simulink model "NN Controlled IM Drive"  (R2020b)
settings: Solver=ode4  StartTime=0.0  StopTime=5  RelTol=1e-3
InitFcn:
  | %clear;
  | %clc;
  | 
  | %Motor Parameters
  | r1 = 1.405;
  | l1  = 0.005839;
  | r2 = 1.395;
  | l2 = 0.005839;
  | Lm = 0.1722;
  | J = 0.0131;
  | 
  | %Motor Rated Values
  | Vrat = 400;
  | frat = 50;
  | 
  | x1 = 2*pi*frat*l1;
  | x2 = 2*pi*frat*l2;
  | Xm = 2*pi*frat*Lm;
  | Prat = 4*1000;
  | Nrat = 1430;
  | P = 4;
  | Ns = 120*frat/P;
  | nrat = Nrat*2*pi/60;
  | ns = Ns*2*pi/60;
  | srat = (Ns-Nrat)/Ns;
  | 
  | E1 = Vrat/sqrt(3); %phase voltage
  | IL = E1/( (r1 + (1i*x1) ) + ( ( (1i*x2) +(r2/srat) )*1i*Xm / ( (1i*Xm) + (1i*x2) + (r2/srat) ) ) );
  | E2 = E1 - (IL*(r1 + (1i*x1) ) );
  | Trat = (3/(ns))*srat*abs(E2)*abs(E2)*r2/((r2*r2) + (srat*srat*x2*x2));
  | %Trat = Prat/nrat;
  | 
  | %System Variables
  | Tsys = (1e-6);
  | Ts = (100e-6);
  | freq = 50;
  | ws = freq*2*pi;
  | 
  | m=1*freq/50;
  | %m = 1 * (freq/50);
  | Vbus = (400*sqrt(2)*2/sqrt(3)) / (1.15);
  | 
  | Vref = (Vbus*sqrt(3)/2) * m;
  | delay = Ts/Tsys;
  | 
  | % Motor Starting Parameters
  | inc_time = 0.1;
  | 
  | %Motor Loading time
  | load_time = 0;
  | 
  | %No. of Hybrid Zones
  | numzones = 3;
  | 
  | %Load ML model Weights
  | 
  | W1R_s1 = readmatrix('Regression Weights\W1_subnet1_tmp_odd_90.xlsx');
  | b1R_s1 = readmatrix('Regression Weights\b1_subnet1_tmp_odd_90.xlsx');
  | W1R_s2 = readmatrix('Regression Weights\W1_subnet2_tmp_odd_90.xlsx');
  | b1R_s2 = readmatrix('Regression Weights\b1_subnet2_tmp_odd_90.xlsx');
  | ... (+47 lines)
undefined symbols (not defined in the file): DiscIntNeverNeededParam
libraries: powerlib x22, simulink x20, pid_lib x4, powerlib_meascontrol x3, simulink_extras x2
(part 2 of 3)

== system NN Controlled IM Drive/Space Vector PWM based VSI /Gating Pulse Generator/Gate Pulse Generator for 1012 Sequence ==
  "S1, S3, S5, sector" : Inport
  AND{,1..5} (6 alike) : Logic  IconShape=distinctive  AllPortsSameDT=off  OutDataTypeStr=boolean
  Constant : Constant  Value=2
  Data Type Conversion : DataTypeConversion
  Demux : Demux
  For Even Sector : Subsystem
  For Odd Sector : Subsystem
  Mod : Math  Operator=mod  SaturateOnIntegerOverflow=on
  Mux : Mux  Inputs=3
  NOT : Logic  Operator=NOT  IconShape=distinctive  AllPortsSameDT=off  OutDataTypeStr=boolean
  OR : Logic  Operator=OR  IconShape=distinctive  AllPortsSameDT=off  OutDataTypeStr=boolean
  OR1 : Logic  Operator=OR  IconShape=distinctive  AllPortsSameDT=off  OutDataTypeStr=boolean
  OR2 : Logic  Operator=OR  IconShape=distinctive  AllPortsSameDT=off  OutDataTypeStr=boolean
  Scope1 : Scope  NumInputPorts=4
  Gate 1 Pulse : Outport
  Gate 3 Pulse : Outport  Port=2
  Gate 5 Pulse : Outport  Port=3
  wires:
  For Odd Sector/3(Gate 5 Pulse) -> AND5/1
  For Odd Sector/1(Gate 1 Pulse) -> AND3/1
  For Even Sector/3(Gate 5 Pulse) -> AND2/1
  For Even Sector/2(Gate 3 Pulse) -> AND1/1
  OR2/1 -> Scope1/3, Gate 5 Pulse/1
  OR1/1 -> Scope1/2, Gate 3 Pulse/1
  Demux/3 -> Mux/3
  For Even Sector/1(Gate 1 Pulse) -> AND/1
  AND4/1 -> OR1/1
  OR/1 -> Scope1/1, Gate 1 Pulse/1
  AND5/1 -> OR2/1
  Demux/2 -> Mux/2
  AND1/1 -> OR1/2
  AND/1 -> OR/2
  Mod/1 -> Data Type Conversion/1
  Demux/4 -> Scope1/4, Mod/1
  Data Type Conversion/1 -> AND3/2, AND4/2, AND5/2, NOT/1
  AND2/1 -> OR2/2
  Demux/1 -> Mux/1
  Mux/1 -> For Even Sector/1("S1, S3, S1"), For Odd Sector/1("S1, S3, S5")
  Constant/1 -> Mod/2
  NOT/1 -> AND/2, AND1/2, AND2/2
  For Odd Sector/2(Gate 3 Pulse) -> AND4/1
  "S1, S3, S5, sector"/1 -> Demux/1
  AND3/1 -> OR/1

== system NN Controlled IM Drive/Space Vector PWM based VSI /Gating Pulse Generator/Gate Pulse Generator for 2721 Sequence ==
  "S1, S3, S5, sector" : Inport
  AND{,1..5} (6 alike) : Logic  IconShape=distinctive  AllPortsSameDT=off  OutDataTypeStr=boolean
  Constant : Constant  Value=2
  Data Type Conversion : DataTypeConversion
  Demux : Demux
  For Even Sector : Subsystem
  For Odd Sector : Subsystem
  Mod : Math  Operator=mod  SaturateOnIntegerOverflow=on
  Mux : Mux  Inputs=3
  NOT : Logic  Operator=NOT  IconShape=distinctive  AllPortsSameDT=off  OutDataTypeStr=boolean
  OR : Logic  Operator=OR  IconShape=distinctive  AllPortsSameDT=off  OutDataTypeStr=boolean
  OR1 : Logic  Operator=OR  IconShape=distinctive  AllPortsSameDT=off  OutDataTypeStr=boolean
  OR2 : Logic  Operator=OR  IconShape=distinctive  AllPortsSameDT=off  OutDataTypeStr=boolean
  Scope1 : Scope  NumInputPorts=4
  Gate 1 Pulse : Outport
  Gate 3 Pulse : Outport  Port=2
  Gate 5 Pulse : Outport  Port=3
  wires:
  For Odd Sector/3(Gate 5 Pulse) -> AND5/1
  For Odd Sector/1(Gate 1 Pulse) -> AND3/1
  For Even Sector/3(Gate 5 Pulse) -> AND2/1
  OR2/1 -> Scope1/3, Gate 5 Pulse/1
  For Even Sector/2(Gate 3 Pulse) -> AND1/1
  OR1/1 -> Scope1/2, Gate 3 Pulse/1
  Demux/3 -> Mux/3
  AND4/1 -> OR1/1
  OR/1 -> Scope1/1, Gate 1 Pulse/1
  AND5/1 -> OR2/1
  Demux/2 -> Mux/2
  For Odd Sector/2(Gate 3 Pulse) -> AND4/1
  AND1/1 -> OR1/2
  AND/1 -> OR/2
  Mod/1 -> Data Type Conversion/1
  Data Type Conversion/1 -> AND3/2, AND4/2, AND5/2, NOT/1
  AND2/1 -> OR2/2
  "S1, S3, S5, sector"/1 -> Demux/1
  AND3/1 -> OR/1
  Demux/4 -> Scope1/4, Mod/1
  Demux/1 -> Mux/1
  Mux/1 -> For Even Sector/1("S1, S3, S5"), For Odd Sector/1("S1, S3, S1")
  Constant/1 -> Mod/2
  NOT/1 -> AND/2, AND1/2, AND2/2
  For Even Sector/1(Gate 1 Pulse) -> AND/1

== system NN Controlled IM Drive/Space Vector PWM based VSI /Gating Pulse Generator/Gate Pulse Generator for 7212 Sequence ==
  "S1, S3, S5, sector" : Inport
  AND{,1..5} (6 alike) : Logic  IconShape=distinctive  AllPortsSameDT=off  OutDataTypeStr=boolean
  Constant : Constant  Value=2
  Data Type Conversion : DataTypeConversion
  Demux : Demux
  For Even Sector : Subsystem
  For Odd Sector : Subsystem
  Mod : Math  Operator=mod  SaturateOnIntegerOverflow=on
  Mux : Mux  Inputs=3
  NOT : Logic  Operator=NOT  IconShape=distinctive  AllPortsSameDT=off  OutDataTypeStr=boolean
  OR : Logic  Operator=OR  IconShape=distinctive  AllPortsSameDT=off  OutDataTypeStr=boolean
  OR1 : Logic  Operator=OR  IconShape=distinctive  AllPortsSameDT=off  OutDataTypeStr=boolean
  OR2 : Logic  Operator=OR  IconShape=distinctive  AllPortsSameDT=off  OutDataTypeStr=boolean
  Scope1 : Scope  NumInputPorts=4
  Gate 1 Pulse : Outport
  Gate 3 Pulse : Outport  Port=2
  Gate 5 Pulse : Outport  Port=3
  wires:
  For Odd Sector/3(Gate 5 Pulse) -> AND5/1
  For Odd Sector/1(Gate 1 Pulse) -> AND3/1
  For Even Sector/3(Gate 5 Pulse) -> AND2/1
  For Even Sector/2(Gate 3 Pulse) -> AND1/1
  OR2/1 -> Scope1/3, Gate 5 Pulse/1
  OR1/1 -> Scope1/2, Gate 3 Pulse/1
  Demux/3 -> Mux/3
  For Even Sector/1(Gate 1 Pulse) -> AND/1
  AND4/1 -> OR1/1
  OR/1 -> Scope1/1, Gate 1 Pulse/1
  AND5/1 -> OR2/1
  Demux/2 -> Mux/2
  AND1/1 -> OR1/2
  AND/1 -> OR/2
  Mod/1 -> Data Type Conversion/1
  Demux/4 -> Scope1/4, Mod/1
  Data Type Conversion/1 -> AND3/2, AND4/2, AND5/2, NOT/1
  AND2/1 -> OR2/2
  Demux/1 -> Mux/1
  Mux/1 -> For Even Sector/1("S1, S3, S1"), For Odd Sector/1("S1, S3, S5")
  Constant/1 -> Mod/2
  NOT/1 -> AND/2, AND1/2, AND2/2
  For Odd Sector/2(Gate 3 Pulse) -> AND4/1
  "S1, S3, S5, sector"/1 -> Demux/1
  AND3/1 -> OR/1

== system NN Controlled IM Drive/Space Vector PWM based VSI /Switching Times and Sector/Angle Calculation1 ==
  freq : Inport
  Delay : Delay  DelayLength=1  InitialCondition=0  UseCircularBuffer=on
  Gain1 : Gain  Gain=Tsys
  MATLAB Function : MATLAB Function  TreatAsAtomicUnit=on
  Scope : Scope
  Zero-Order Hold : ZeroOrderHold  SampleTime=Ts
  w : Gain  Gain=2*pi
  Angle : Outport
  tag scope: wt=global
  wires:
  freq/1 -> w/1, Scope/1
  Gain1/1 -> MATLAB Function/2(wTs)
  Zero-Order Hold/1 -> Angle/1
  Delay/1 -> MATLAB Function/1(wold)
  MATLAB Function/1(wnew) -> Delay/1, Zero-Order Hold/1, [wt]
  w/1 -> Gain1/1

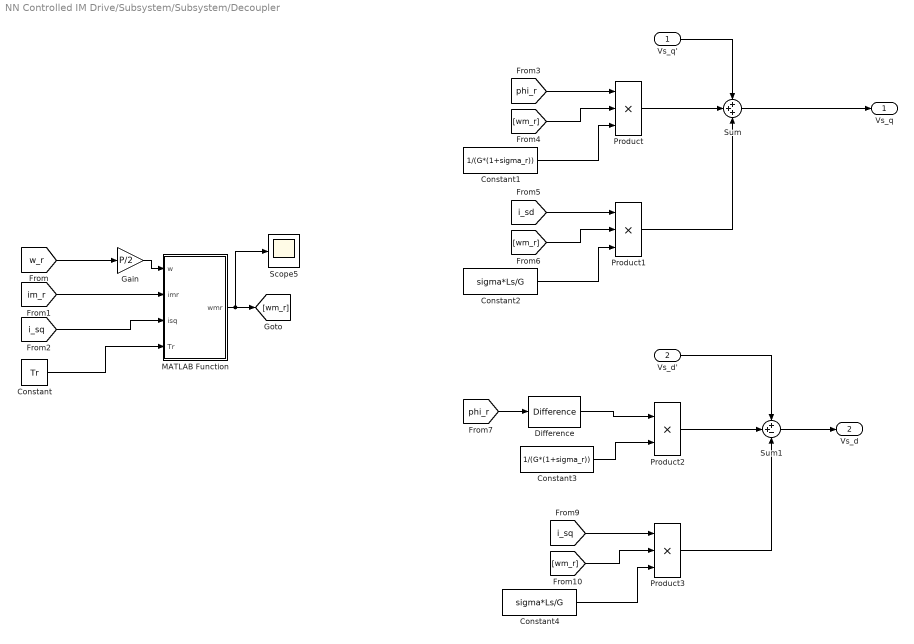
== system NN Controlled IM Drive/Subsystem/Subsystem/Decoupler ==
  Vs_q' : Inport
  Vs_d' : Inport  Port=2
  Constant : Constant  Value=Tr
  Constant1 : Constant  Value=1/(G*(1+sigma_r))
  Constant2 : Constant  Value=sigma*Ls/G
  Constant3 : Constant  Value=1/(G*(1+sigma_r))
  Constant4 : Constant  Value=sigma*Ls/G
  Difference : simulink/Discrete/Difference  ICPrevInput=0.0  OutMin=[]  OutMax=[]  OutDataType=fixdt(1, 16)  OutScaling=2^-10  DoSatur=off
  Gain : Gain  Gain=P/2
  MATLAB Function : MATLAB Function  TreatAsAtomicUnit=on
  Product : Product  Inputs=3
  Product1 : Product  Inputs=3
  Product2 : Product
  Product3 : Product  Inputs=3
  Scope5 : Scope
  Sum : Sum  Inputs=+++
  Sum1 : Sum  Inputs=++-
  Vs_q : Outport
  Vs_d : Outport  Port=2
  wires:
  [im_r] -> MATLAB Function/2(imr)
  [i_sq] -> MATLAB Function/3(isq)
  Constant/1 -> MATLAB Function/4(Tr)
  MATLAB Function/1(wmr) -> Scope5/1, [wm_r]
  [phi_r] -> Product/1
  [wm_r] -> Product/2
  Constant1/1 -> Product/3
  Vs_q'/1 -> Sum/1
  Product/1 -> Sum/2
  Constant2/1 -> Product1/3
  [wm_r] -> Product1/2
  [i_sd] -> Product1/1
  Product1/1 -> Sum/3
  Sum/1 -> Vs_q/1
  Product3/1 -> Sum1/3
  [i_sq] -> Product3/1
  [wm_r] -> Product3/2
  Constant4/1 -> Product3/3
  Difference/1 -> Product2/1
  Vs_d'/1 -> Sum1/1
  Sum1/1 -> Vs_d/1
  [phi_r] -> Difference/1
  Constant3/1 -> Product2/2
  [w_r] -> Gain/1
  Gain/1 -> MATLAB Function/1(w)
  Product2/1 -> Sum1/2

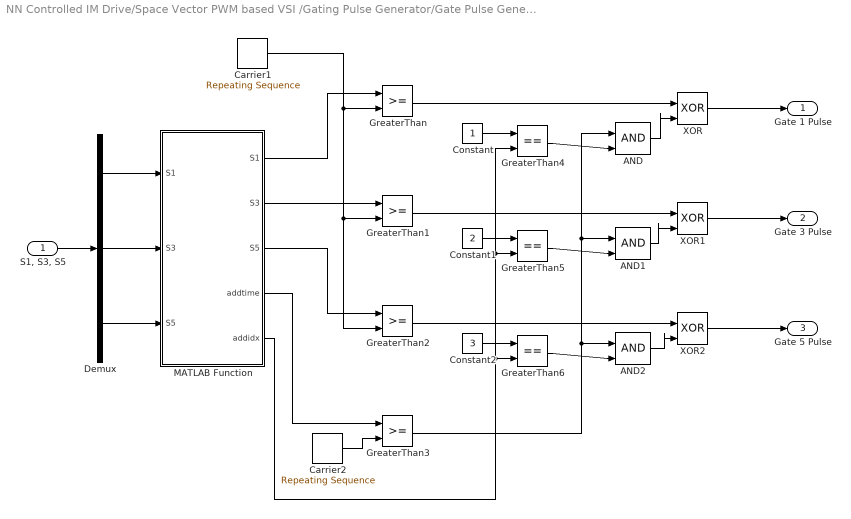
== system NN Controlled IM Drive/Space Vector PWM based VSI /Gating Pulse Generator/Gate Pulse Generator for 0121 Sequence/For Even Sector ==
  "S1, S3, S5" : Inport
  AND : Logic  IconShape=distinctive  AllPortsSameDT=off  OutDataTypeStr=boolean
  AND1 : Logic  IconShape=distinctive  AllPortsSameDT=off  OutDataTypeStr=boolean
  AND2 : Logic  IconShape=distinctive  AllPortsSameDT=off  OutDataTypeStr=boolean
  Carrier1 : simulink/Sources/Repeating Sequence  rep_seq_t=[0 Ts/2 Ts]  rep_seq_y=[0 Ts-(1e-16) 0]
  Carrier2 : simulink/Sources/Repeating Sequence  rep_seq_t=[0 Ts/2 Ts]  rep_seq_y=[Ts-(1e-16) 0 Ts-(1e-16)]
  Constant : Constant
  Constant1 : Constant  Value=2
  Constant2 : Constant  Value=3
  Demux : Demux  Outputs=3
  GreaterThan{,1..3} (4 alike) : RelationalOperator  OutDataTypeStr=boolean  RndMeth=Simplest
  GreaterThan4 : RelationalOperator  Operator===  OutDataTypeStr=boolean  RndMeth=Simplest
  GreaterThan5 : RelationalOperator  Operator===  OutDataTypeStr=boolean  RndMeth=Simplest
  GreaterThan6 : RelationalOperator  Operator===  OutDataTypeStr=boolean  RndMeth=Simplest
  MATLAB Function : MATLAB Function  TreatAsAtomicUnit=on
  XOR : Logic  Operator=XOR  IconShape=distinctive  AllPortsSameDT=off  OutDataTypeStr=boolean
  XOR1 : Logic  Operator=XOR  IconShape=distinctive  AllPortsSameDT=off  OutDataTypeStr=boolean
  XOR2 : Logic  Operator=XOR  IconShape=distinctive  AllPortsSameDT=off  OutDataTypeStr=boolean
  Gate 1 Pulse : Outport
  Gate 3 Pulse : Outport  Port=2
  Gate 5 Pulse : Outport  Port=3
  wires:
  Demux/3 -> MATLAB Function/3("S5 ")
  Demux/1 -> MATLAB Function/1("S1 ")
  "S1, S3, S5"/1 -> Demux/1
  Demux/2 -> MATLAB Function/2("S3 ")
  MATLAB Function/5(addidx) -> GreaterThan6/2, GreaterThan5/2, GreaterThan4/2
  Constant1/1 -> GreaterThan5/1
  Constant/1 -> GreaterThan4/1
  XOR1/1 -> Gate 3 Pulse/1
  GreaterThan6/1 -> AND2/2
  Constant2/1 -> GreaterThan6/1
  GreaterThan5/1 -> AND1/2
  AND/1 -> XOR/2
  AND2/1 -> XOR2/2
  GreaterThan2/1 -> XOR2/1
  MATLAB Function/1(S1) -> GreaterThan/1
  GreaterThan/1 -> XOR/1
  MATLAB Function/4(addtime) -> GreaterThan3/1
  GreaterThan4/1 -> AND/2
  XOR2/1 -> Gate 5 Pulse/1
  GreaterThan3/1 -> AND/1, AND1/1, AND2/1
  AND1/1 -> XOR1/2
  MATLAB Function/3(S5) -> GreaterThan2/1
  MATLAB Function/2(S3) -> GreaterThan1/1
  XOR/1 -> Gate 1 Pulse/1
  Carrier1/1 -> GreaterThan/2, GreaterThan1/2, GreaterThan2/2
  GreaterThan1/1 -> XOR1/1
  Carrier2/1 -> GreaterThan3/2

== system NN Controlled IM Drive/Space Vector PWM based VSI /Gating Pulse Generator/Gate Pulse Generator for 0121 Sequence/For Odd Sector ==
  "S1, S3, S5" : Inport
  AND : Logic  IconShape=distinctive  AllPortsSameDT=off  OutDataTypeStr=boolean
  AND1 : Logic  IconShape=distinctive  AllPortsSameDT=off  OutDataTypeStr=boolean
  AND2 : Logic  IconShape=distinctive  AllPortsSameDT=off  OutDataTypeStr=boolean
  Carrier1 : simulink/Sources/Repeating Sequence  rep_seq_t=[0 Ts/2 Ts]  rep_seq_y=[Ts-(1e-16) 0 Ts-(1e-16)]
  Constant : Constant
  Constant1 : Constant  Value=2
  Constant2 : Constant  Value=3
  Demux : Demux  Outputs=3
  GreaterThan{,1..3} (4 alike) : RelationalOperator  OutDataTypeStr=boolean  RndMeth=Simplest
  GreaterThan4 : RelationalOperator  Operator===  OutDataTypeStr=boolean  RndMeth=Simplest
  GreaterThan5 : RelationalOperator  Operator===  OutDataTypeStr=boolean  RndMeth=Simplest
  GreaterThan6 : RelationalOperator  Operator===  OutDataTypeStr=boolean  RndMeth=Simplest
  MATLAB Function : MATLAB Function  TreatAsAtomicUnit=on
  XOR : Logic  Operator=XOR  IconShape=distinctive  AllPortsSameDT=off  OutDataTypeStr=boolean
  XOR1 : Logic  Operator=XOR  IconShape=distinctive  AllPortsSameDT=off  OutDataTypeStr=boolean
  XOR2 : Logic  Operator=XOR  IconShape=distinctive  AllPortsSameDT=off  OutDataTypeStr=boolean
  Gate 1 Pulse : Outport
  Gate 3 Pulse : Outport  Port=2
  Gate 5 Pulse : Outport  Port=3
  wires:
  "S1, S3, S5"/1 -> Demux/1
  Demux/1 -> MATLAB Function/1("S1 ")
  Demux/2 -> MATLAB Function/2("S3 ")
  Demux/3 -> MATLAB Function/3("S5 ")
  MATLAB Function/1(S1) -> GreaterThan/1
  Carrier1/1 -> GreaterThan/2, GreaterThan1/2, GreaterThan3/2, GreaterThan2/2
  MATLAB Function/2(S3) -> GreaterThan1/1
  MATLAB Function/3(S5) -> GreaterThan2/1
  MATLAB Function/4(subtime) -> GreaterThan3/1
  MATLAB Function/5(subidx) -> GreaterThan6/2, GreaterThan5/2, GreaterThan4/2
  Constant/1 -> GreaterThan4/1
  Constant1/1 -> GreaterThan5/1
  Constant2/1 -> GreaterThan6/1
  GreaterThan4/1 -> AND/2
  GreaterThan5/1 -> AND1/2
  GreaterThan6/1 -> AND2/2
  GreaterThan3/1 -> AND/1, AND1/1, AND2/1
  AND/1 -> XOR/2
  GreaterThan/1 -> XOR/1
  GreaterThan1/1 -> XOR1/1
  AND1/1 -> XOR1/2
  GreaterThan2/1 -> XOR2/1
  AND2/1 -> XOR2/2
  XOR/1 -> Gate 1 Pulse/1
  XOR1/1 -> Gate 3 Pulse/1
  XOR2/1 -> Gate 5 Pulse/1

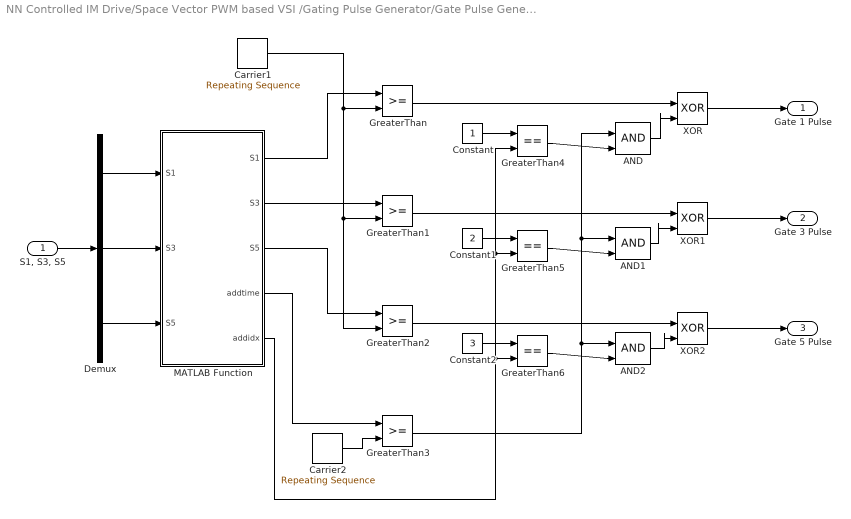
== system NN Controlled IM Drive/Space Vector PWM based VSI /Gating Pulse Generator/Gate Pulse Generator for 0127 Sequence 1/For Even Sector ==
  "S1, S3, S5" : Inport
  AND : Logic  IconShape=distinctive  AllPortsSameDT=off  OutDataTypeStr=boolean
  AND1 : Logic  IconShape=distinctive  AllPortsSameDT=off  OutDataTypeStr=boolean
  AND2 : Logic  IconShape=distinctive  AllPortsSameDT=off  OutDataTypeStr=boolean
  Carrier1 : simulink/Sources/Repeating Sequence  rep_seq_t=[0 Ts/2 Ts]  rep_seq_y=[Ts-(1e-16) 0 Ts-(1e-16)]
  Carrier2 : simulink/Sources/Repeating Sequence  rep_seq_t=[0 Ts/2 Ts]  rep_seq_y=[0 Ts-(1e-16) 0]
  Constant : Constant
  Constant1 : Constant  Value=2
  Constant2 : Constant  Value=3
  Demux : Demux  Outputs=3
  GreaterThan{,1..3} (4 alike) : RelationalOperator  OutDataTypeStr=boolean  RndMeth=Simplest
  GreaterThan4 : RelationalOperator  Operator===  OutDataTypeStr=boolean  RndMeth=Simplest
  GreaterThan5 : RelationalOperator  Operator===  OutDataTypeStr=boolean  RndMeth=Simplest
  GreaterThan6 : RelationalOperator  Operator===  OutDataTypeStr=boolean  RndMeth=Simplest
  MATLAB Function : MATLAB Function  TreatAsAtomicUnit=on
  XOR : Logic  Operator=XOR  IconShape=distinctive  AllPortsSameDT=off  OutDataTypeStr=boolean
  XOR1 : Logic  Operator=XOR  IconShape=distinctive  AllPortsSameDT=off  OutDataTypeStr=boolean
  XOR2 : Logic  Operator=XOR  IconShape=distinctive  AllPortsSameDT=off  OutDataTypeStr=boolean
  Gate 1 Pulse : Outport
  Gate 3 Pulse : Outport  Port=2
  Gate 5 Pulse : Outport  Port=3
  wires:
  AND/1 -> XOR/2
  GreaterThan2/1 -> XOR2/1
  "S1, S3, S5"/1 -> Demux/1
  MATLAB Function/1(S1) -> GreaterThan/1
  Demux/1 -> MATLAB Function/1("S1 ")
  Demux/2 -> MATLAB Function/2("S3 ")
  Demux/3 -> MATLAB Function/3("S5 ")
  Carrier2/1 -> GreaterThan3/2
  XOR2/1 -> Gate 5 Pulse/1
  GreaterThan6/1 -> AND2/2
  GreaterThan1/1 -> XOR1/1
  GreaterThan3/1 -> AND/1, AND1/1, AND2/1
  GreaterThan4/1 -> AND/2
  Constant2/1 -> GreaterThan6/1
  AND1/1 -> XOR1/2
  MATLAB Function/2(S3) -> GreaterThan1/1
  MATLAB Function/4(addtime) -> GreaterThan3/1
  XOR/1 -> Gate 1 Pulse/1
  Carrier1/1 -> GreaterThan/2, GreaterThan1/2, GreaterThan2/2
  Constant/1 -> GreaterThan4/1
  MATLAB Function/5(addidx) -> GreaterThan6/2, GreaterThan5/2, GreaterThan4/2
  GreaterThan5/1 -> AND1/2
  GreaterThan/1 -> XOR/1
  XOR1/1 -> Gate 3 Pulse/1
  MATLAB Function/3(S5) -> GreaterThan2/1
  AND2/1 -> XOR2/2
  Constant1/1 -> GreaterThan5/1

== system NN Controlled IM Drive/Space Vector PWM based VSI /Gating Pulse Generator/Gate Pulse Generator for 0127 Sequence 1/For Odd Sector ==
  "S1, S3, S1" : Inport
  AND3 : Logic  IconShape=distinctive  AllPortsSameDT=off  OutDataTypeStr=boolean
  AND4 : Logic  IconShape=distinctive  AllPortsSameDT=off  OutDataTypeStr=boolean
  AND5 : Logic  IconShape=distinctive  AllPortsSameDT=off  OutDataTypeStr=boolean
  Carrier3 : simulink/Sources/Repeating Sequence  rep_seq_t=[0 Ts/2 Ts]  rep_seq_y=[0 Ts-(1e-16) 0]
  Constant3 : Constant
  Constant4 : Constant  Value=2
  Constant5 : Constant  Value=3
  Demux1 : Demux  Outputs=3
  GreaterThan{7..10} (4 alike) : RelationalOperator  OutDataTypeStr=boolean  RndMeth=Simplest
  GreaterThan11 : RelationalOperator  Operator===  OutDataTypeStr=boolean  RndMeth=Simplest
  GreaterThan12 : RelationalOperator  Operator===  OutDataTypeStr=boolean  RndMeth=Simplest
  GreaterThan13 : RelationalOperator  Operator===  OutDataTypeStr=boolean  RndMeth=Simplest
  MATLAB Function1 : MATLAB Function  TreatAsAtomicUnit=on
  XOR3 : Logic  Operator=XOR  IconShape=distinctive  AllPortsSameDT=off  OutDataTypeStr=boolean
  XOR4 : Logic  Operator=XOR  IconShape=distinctive  AllPortsSameDT=off  OutDataTypeStr=boolean
  XOR5 : Logic  Operator=XOR  IconShape=distinctive  AllPortsSameDT=off  OutDataTypeStr=boolean
  Gate 1 Pulse1 : Outport
  Gate 3 Pulse1 : Outport  Port=2
  Gate 5 Pulse1 : Outport  Port=3
  wires:
  GreaterThan12/1 -> AND4/2
  GreaterThan9/1 -> XOR5/1
  Constant4/1 -> GreaterThan12/1
  MATLAB Function1/3(S5) -> GreaterThan9/1
  GreaterThan10/1 -> AND3/1, AND4/1, AND5/1
  MATLAB Function1/5(subidx) -> GreaterThan13/2, GreaterThan12/2, GreaterThan11/2
  MATLAB Function1/2(S3) -> GreaterThan8/1
  AND5/1 -> XOR5/2
  Demux1/2 -> MATLAB Function1/2("S3 ")
  AND4/1 -> XOR4/2
  Demux1/1 -> MATLAB Function1/1("S1 ")
  GreaterThan11/1 -> AND3/2
  AND3/1 -> XOR3/2
  MATLAB Function1/1(S1) -> GreaterThan7/1
  GreaterThan8/1 -> XOR4/1
  GreaterThan13/1 -> AND5/2
  Constant5/1 -> GreaterThan13/1
  GreaterThan7/1 -> XOR3/1
  XOR4/1 -> Gate 3 Pulse1/1
  Demux1/3 -> MATLAB Function1/3("S5 ")
  XOR5/1 -> Gate 5 Pulse1/1
  Constant3/1 -> GreaterThan11/1
  XOR3/1 -> Gate 1 Pulse1/1
  "S1, S3, S1"/1 -> Demux1/1
  Carrier3/1 -> GreaterThan7/2, GreaterThan8/2, GreaterThan10/2, GreaterThan9/2
  MATLAB Function1/4(subtime) -> GreaterThan10/1

== system NN Controlled IM Drive/Space Vector PWM based VSI /Gating Pulse Generator/Gate Pulse Generator for 1012 Sequence/For Even Sector ==
  "S1, S3, S1" : Inport
  AND3 : Logic  IconShape=distinctive  AllPortsSameDT=off  OutDataTypeStr=boolean
  AND4 : Logic  IconShape=distinctive  AllPortsSameDT=off  OutDataTypeStr=boolean
  AND5 : Logic  IconShape=distinctive  AllPortsSameDT=off  OutDataTypeStr=boolean
  Carrier2 : simulink/Sources/Repeating Sequence  rep_seq_t=[0 Ts/2 Ts]  rep_seq_y=[0 Ts-(1e-16) 0]
  Constant3 : Constant
  Constant4 : Constant  Value=2
  Constant5 : Constant  Value=3
  Demux1 : Demux  Outputs=3
  GreaterThan{7..10} (4 alike) : RelationalOperator  OutDataTypeStr=boolean  RndMeth=Simplest
  GreaterThan11 : RelationalOperator  Operator===  OutDataTypeStr=boolean  RndMeth=Simplest
  GreaterThan12 : RelationalOperator  Operator===  OutDataTypeStr=boolean  RndMeth=Simplest
  GreaterThan13 : RelationalOperator  Operator===  OutDataTypeStr=boolean  RndMeth=Simplest
  MATLAB Function1 : MATLAB Function  TreatAsAtomicUnit=on
  XOR3 : Logic  Operator=XOR  IconShape=distinctive  AllPortsSameDT=off  OutDataTypeStr=boolean
  XOR4 : Logic  Operator=XOR  IconShape=distinctive  AllPortsSameDT=off  OutDataTypeStr=boolean
  XOR5 : Logic  Operator=XOR  IconShape=distinctive  AllPortsSameDT=off  OutDataTypeStr=boolean
  Gate 1 Pulse : Outport
  Gate 3 Pulse : Outport  Port=2
  Gate 5 Pulse : Outport  Port=3
  wires:
  XOR3/1 -> Gate 1 Pulse/1
  XOR5/1 -> Gate 5 Pulse/1
  Demux1/3 -> MATLAB Function1/3("S5 ")
  GreaterThan7/1 -> XOR3/1
  GreaterThan11/1 -> AND3/2
  Demux1/2 -> MATLAB Function1/2("S3 ")
  GreaterThan8/1 -> XOR4/1
  XOR4/1 -> Gate 3 Pulse/1
  AND4/1 -> XOR4/2
  AND3/1 -> XOR3/2
  MATLAB Function1/4(subtime) -> GreaterThan10/1
  AND5/1 -> XOR5/2
  GreaterThan13/1 -> AND5/2
  Constant5/1 -> GreaterThan13/1
  Constant3/1 -> GreaterThan11/1
  MATLAB Function1/2(S3) -> GreaterThan8/1
  Demux1/1 -> MATLAB Function1/1("S1 ")
  MATLAB Function1/5(subidx) -> GreaterThan13/2, GreaterThan12/2, GreaterThan11/2
  MATLAB Function1/3(S5) -> GreaterThan9/1
  MATLAB Function1/1(S1) -> GreaterThan7/1
  GreaterThan10/1 -> AND3/1, AND4/1, AND5/1
  Constant4/1 -> GreaterThan12/1
  GreaterThan9/1 -> XOR5/1
  "S1, S3, S1"/1 -> Demux1/1
  Carrier2/1 -> GreaterThan7/2, GreaterThan8/2, GreaterThan10/2, GreaterThan9/2
  GreaterThan12/1 -> AND4/2

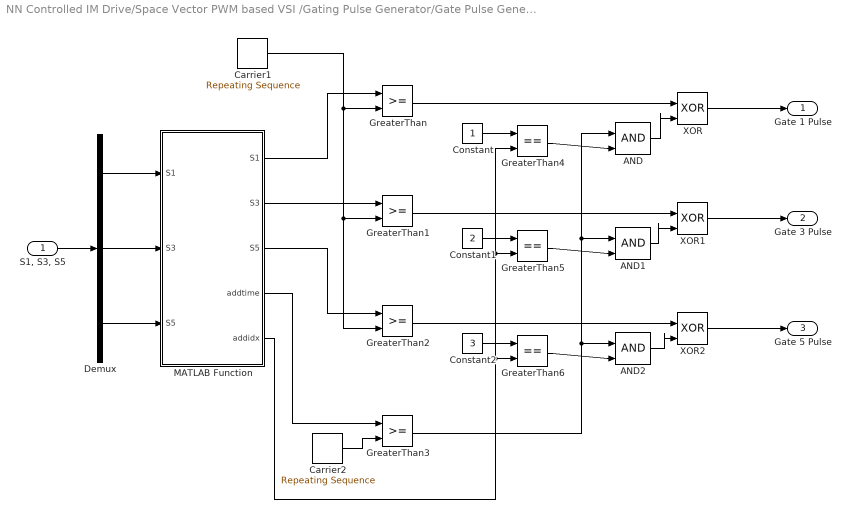
== system NN Controlled IM Drive/Space Vector PWM based VSI /Gating Pulse Generator/Gate Pulse Generator for 1012 Sequence/For Odd Sector ==
  "S1, S3, S5" : Inport
  AND : Logic  IconShape=distinctive  AllPortsSameDT=off  OutDataTypeStr=boolean
  AND1 : Logic  IconShape=distinctive  AllPortsSameDT=off  OutDataTypeStr=boolean
  AND2 : Logic  IconShape=distinctive  AllPortsSameDT=off  OutDataTypeStr=boolean
  Carrier1 : simulink/Sources/Repeating Sequence  rep_seq_t=[0 Ts/2 Ts]  rep_seq_y=[Ts-(1e-16) 0 Ts-(1e-16)]
  Carrier2 : simulink/Sources/Repeating Sequence  rep_seq_t=[0 Ts/2 Ts]  rep_seq_y=[0 Ts-(1e-16) 0]
  Constant : Constant
  Constant1 : Constant  Value=2
  Constant2 : Constant  Value=3
  Demux : Demux  Outputs=3
  GreaterThan{,1..3} (4 alike) : RelationalOperator  OutDataTypeStr=boolean  RndMeth=Simplest
  GreaterThan4 : RelationalOperator  Operator===  OutDataTypeStr=boolean  RndMeth=Simplest
  GreaterThan5 : RelationalOperator  Operator===  OutDataTypeStr=boolean  RndMeth=Simplest
  GreaterThan6 : RelationalOperator  Operator===  OutDataTypeStr=boolean  RndMeth=Simplest
  MATLAB Function : MATLAB Function  TreatAsAtomicUnit=on
  XOR : Logic  Operator=XOR  IconShape=distinctive  AllPortsSameDT=off  OutDataTypeStr=boolean
  XOR1 : Logic  Operator=XOR  IconShape=distinctive  AllPortsSameDT=off  OutDataTypeStr=boolean
  XOR2 : Logic  Operator=XOR  IconShape=distinctive  AllPortsSameDT=off  OutDataTypeStr=boolean
  Gate 1 Pulse : Outport
  Gate 3 Pulse : Outport  Port=2
  Gate 5 Pulse : Outport  Port=3
  wires:
  Carrier1/1 -> GreaterThan/2, GreaterThan1/2, GreaterThan2/2
  MATLAB Function/2(S3) -> GreaterThan1/1
  XOR/1 -> Gate 1 Pulse/1
  MATLAB Function/3(S5) -> GreaterThan2/1
  Constant/1 -> GreaterThan4/1
  MATLAB Function/4(addtime) -> GreaterThan3/1
  GreaterThan/1 -> XOR/1
  AND1/1 -> XOR1/2
  GreaterThan3/1 -> AND/1, AND1/1, AND2/1
  GreaterThan1/1 -> XOR1/1
  XOR2/1 -> Gate 5 Pulse/1
  GreaterThan4/1 -> AND/2
  MATLAB Function/1(S1) -> GreaterThan/1
  Carrier2/1 -> GreaterThan3/2
  GreaterThan2/1 -> XOR2/1
  GreaterThan5/1 -> AND1/2
  Constant2/1 -> GreaterThan6/1
  "S1, S3, S5"/1 -> Demux/1
  AND/1 -> XOR/2
  AND2/1 -> XOR2/2
  Constant1/1 -> GreaterThan5/1
  XOR1/1 -> Gate 3 Pulse/1
  MATLAB Function/5(addidx) -> GreaterThan6/2, GreaterThan5/2, GreaterThan4/2
  Demux/3 -> MATLAB Function/3("S5 ")
  Demux/1 -> MATLAB Function/1("S1 ")
  Demux/2 -> MATLAB Function/2("S3 ")
  GreaterThan6/1 -> AND2/2

== system NN Controlled IM Drive/Space Vector PWM based VSI /Gating Pulse Generator/Gate Pulse Generator for 2721 Sequence/For Even Sector ==
  "S1, S3, S5" : Inport
  AND : Logic  IconShape=distinctive  AllPortsSameDT=off  OutDataTypeStr=boolean
  AND1 : Logic  IconShape=distinctive  AllPortsSameDT=off  OutDataTypeStr=boolean
  AND2 : Logic  IconShape=distinctive  AllPortsSameDT=off  OutDataTypeStr=boolean
  Carrier1 : simulink/Sources/Repeating Sequence  rep_seq_t=[0 Ts/2 Ts]  rep_seq_y=[Ts-(1e-16) 0 Ts-(1e-16)]
  Carrier2 : simulink/Sources/Repeating Sequence  rep_seq_t=[0 Ts/2 Ts]  rep_seq_y=[0 Ts-(1e-16) 0]
  Constant : Constant
  Constant1 : Constant  Value=2
  Constant2 : Constant  Value=3
  Demux : Demux  Outputs=3
  GreaterThan{,1..3} (4 alike) : RelationalOperator  OutDataTypeStr=boolean  RndMeth=Simplest
  GreaterThan4 : RelationalOperator  Operator===  OutDataTypeStr=boolean  RndMeth=Simplest
  GreaterThan5 : RelationalOperator  Operator===  OutDataTypeStr=boolean  RndMeth=Simplest
  GreaterThan6 : RelationalOperator  Operator===  OutDataTypeStr=boolean  RndMeth=Simplest
  MATLAB Function : MATLAB Function  TreatAsAtomicUnit=on
  XOR : Logic  Operator=XOR  IconShape=distinctive  AllPortsSameDT=off  OutDataTypeStr=boolean
  XOR1 : Logic  Operator=XOR  IconShape=distinctive  AllPortsSameDT=off  OutDataTypeStr=boolean
  XOR2 : Logic  Operator=XOR  IconShape=distinctive  AllPortsSameDT=off  OutDataTypeStr=boolean
  Gate 1 Pulse : Outport
  Gate 3 Pulse : Outport  Port=2
  Gate 5 Pulse : Outport  Port=3
  wires:
  AND/1 -> XOR/2
  GreaterThan2/1 -> XOR2/1
  "S1, S3, S5"/1 -> Demux/1
  MATLAB Function/1(S1) -> GreaterThan/1
  Demux/1 -> MATLAB Function/1("S1 ")
  Demux/2 -> MATLAB Function/2("S3 ")
  Demux/3 -> MATLAB Function/3("S5 ")
  Carrier2/1 -> GreaterThan3/2
  XOR2/1 -> Gate 5 Pulse/1
  GreaterThan6/1 -> AND2/2
  GreaterThan1/1 -> XOR1/1
  GreaterThan3/1 -> AND/1, AND1/1, AND2/1
  GreaterThan4/1 -> AND/2
  Constant2/1 -> GreaterThan6/1
  AND1/1 -> XOR1/2
  MATLAB Function/2(S3) -> GreaterThan1/1
  MATLAB Function/4(addtime) -> GreaterThan3/1
  XOR/1 -> Gate 1 Pulse/1
  Carrier1/1 -> GreaterThan/2, GreaterThan1/2, GreaterThan2/2
  Constant/1 -> GreaterThan4/1
  MATLAB Function/5(addidx) -> GreaterThan6/2, GreaterThan5/2, GreaterThan4/2
  GreaterThan5/1 -> AND1/2
  GreaterThan/1 -> XOR/1
  XOR1/1 -> Gate 3 Pulse/1
  MATLAB Function/3(S5) -> GreaterThan2/1
  AND2/1 -> XOR2/2
  Constant1/1 -> GreaterThan5/1

== system NN Controlled IM Drive/Space Vector PWM based VSI /Gating Pulse Generator/Gate Pulse Generator for 2721 Sequence/For Odd Sector ==
  "S1, S3, S1" : Inport
  AND3 : Logic  IconShape=distinctive  AllPortsSameDT=off  OutDataTypeStr=boolean
  AND4 : Logic  IconShape=distinctive  AllPortsSameDT=off  OutDataTypeStr=boolean
  AND5 : Logic  IconShape=distinctive  AllPortsSameDT=off  OutDataTypeStr=boolean
  Carrier3 : simulink/Sources/Repeating Sequence  rep_seq_t=[0 Ts/2 Ts]  rep_seq_y=[0 Ts-(1e-16) 0]
  Constant3 : Constant
  Constant4 : Constant  Value=2
  Constant5 : Constant  Value=3
  Demux1 : Demux  Outputs=3
  GreaterThan{7..10} (4 alike) : RelationalOperator  OutDataTypeStr=boolean  RndMeth=Simplest
  GreaterThan11 : RelationalOperator  Operator===  OutDataTypeStr=boolean  RndMeth=Simplest
  GreaterThan12 : RelationalOperator  Operator===  OutDataTypeStr=boolean  RndMeth=Simplest
  GreaterThan13 : RelationalOperator  Operator===  OutDataTypeStr=boolean  RndMeth=Simplest
  MATLAB Function1 : MATLAB Function  TreatAsAtomicUnit=on
  XOR3 : Logic  Operator=XOR  IconShape=distinctive  AllPortsSameDT=off  OutDataTypeStr=boolean
  XOR4 : Logic  Operator=XOR  IconShape=distinctive  AllPortsSameDT=off  OutDataTypeStr=boolean
  XOR5 : Logic  Operator=XOR  IconShape=distinctive  AllPortsSameDT=off  OutDataTypeStr=boolean
  Gate 1 Pulse : Outport
  Gate 3 Pulse : Outport  Port=2
  Gate 5 Pulse : Outport  Port=3
  wires:
  GreaterThan12/1 -> AND4/2
  GreaterThan9/1 -> XOR5/1
  Constant4/1 -> GreaterThan12/1
  MATLAB Function1/3(S5) -> GreaterThan9/1
  GreaterThan10/1 -> AND3/1, AND4/1, AND5/1
  MATLAB Function1/5(subidx) -> GreaterThan13/2, GreaterThan12/2, GreaterThan11/2
  MATLAB Function1/2(S3) -> GreaterThan8/1
  AND5/1 -> XOR5/2
  Demux1/2 -> MATLAB Function1/2("S3 ")
  AND4/1 -> XOR4/2
  Demux1/1 -> MATLAB Function1/1("S1 ")
  GreaterThan11/1 -> AND3/2
  AND3/1 -> XOR3/2
  MATLAB Function1/1(S1) -> GreaterThan7/1
  GreaterThan8/1 -> XOR4/1
  GreaterThan13/1 -> AND5/2
  Constant5/1 -> GreaterThan13/1
  GreaterThan7/1 -> XOR3/1
  XOR4/1 -> Gate 3 Pulse/1
  Demux1/3 -> MATLAB Function1/3("S5 ")
  XOR5/1 -> Gate 5 Pulse/1
  Constant3/1 -> GreaterThan11/1
  XOR3/1 -> Gate 1 Pulse/1
  "S1, S3, S1"/1 -> Demux1/1
  Carrier3/1 -> GreaterThan7/2, GreaterThan8/2, GreaterThan10/2, GreaterThan9/2
  MATLAB Function1/4(subtime) -> GreaterThan10/1

== system NN Controlled IM Drive/Space Vector PWM based VSI /Gating Pulse Generator/Gate Pulse Generator for 7212 Sequence/For Even Sector ==
  "S1, S3, S1" : Inport
  AND3 : Logic  IconShape=distinctive  AllPortsSameDT=off  OutDataTypeStr=boolean
  AND4 : Logic  IconShape=distinctive  AllPortsSameDT=off  OutDataTypeStr=boolean
  AND5 : Logic  IconShape=distinctive  AllPortsSameDT=off  OutDataTypeStr=boolean
  Carrier3 : simulink/Sources/Repeating Sequence  rep_seq_t=[0 Ts/2 Ts]  rep_seq_y=[Ts-(1e-16) 0 Ts-(1e-16)]
  Constant3 : Constant
  Constant4 : Constant  Value=2
  Constant5 : Constant  Value=3
  Demux1 : Demux  Outputs=3
  GreaterThan{7..10} (4 alike) : RelationalOperator  OutDataTypeStr=boolean  RndMeth=Simplest
  GreaterThan11 : RelationalOperator  Operator===  OutDataTypeStr=boolean  RndMeth=Simplest
  GreaterThan12 : RelationalOperator  Operator===  OutDataTypeStr=boolean  RndMeth=Simplest
  GreaterThan13 : RelationalOperator  Operator===  OutDataTypeStr=boolean  RndMeth=Simplest
  MATLAB Function1 : MATLAB Function  TreatAsAtomicUnit=on
  XOR3 : Logic  Operator=XOR  IconShape=distinctive  AllPortsSameDT=off  OutDataTypeStr=boolean
  XOR4 : Logic  Operator=XOR  IconShape=distinctive  AllPortsSameDT=off  OutDataTypeStr=boolean
  XOR5 : Logic  Operator=XOR  IconShape=distinctive  AllPortsSameDT=off  OutDataTypeStr=boolean
  Gate 1 Pulse : Outport
  Gate 3 Pulse : Outport  Port=2
  Gate 5 Pulse : Outport  Port=3
  wires:
  XOR3/1 -> Gate 1 Pulse/1
  XOR5/1 -> Gate 5 Pulse/1
  Demux1/3 -> MATLAB Function1/3("S5 ")
  GreaterThan7/1 -> XOR3/1
  GreaterThan11/1 -> AND3/2
  Demux1/2 -> MATLAB Function1/2("S3 ")
  GreaterThan8/1 -> XOR4/1
  XOR4/1 -> Gate 3 Pulse/1
  AND4/1 -> XOR4/2
  AND3/1 -> XOR3/2
  MATLAB Function1/4(subtime) -> GreaterThan10/1
  AND5/1 -> XOR5/2
  GreaterThan13/1 -> AND5/2
  Constant5/1 -> GreaterThan13/1
  Constant3/1 -> GreaterThan11/1
  MATLAB Function1/2(S3) -> GreaterThan8/1
  Demux1/1 -> MATLAB Function1/1("S1 ")
  MATLAB Function1/5(subidx) -> GreaterThan13/2, GreaterThan12/2, GreaterThan11/2
  MATLAB Function1/3(S5) -> GreaterThan9/1
  MATLAB Function1/1(S1) -> GreaterThan7/1
  GreaterThan10/1 -> AND3/1, AND4/1, AND5/1
  Constant4/1 -> GreaterThan12/1
  GreaterThan9/1 -> XOR5/1
  "S1, S3, S1"/1 -> Demux1/1
  Carrier3/1 -> GreaterThan7/2, GreaterThan8/2, GreaterThan10/2, GreaterThan9/2
  GreaterThan12/1 -> AND4/2

== system NN Controlled IM Drive/Space Vector PWM based VSI /Gating Pulse Generator/Gate Pulse Generator for 7212 Sequence/For Odd Sector ==
  "S1, S3, S5" : Inport
  AND : Logic  IconShape=distinctive  AllPortsSameDT=off  OutDataTypeStr=boolean
  AND1 : Logic  IconShape=distinctive  AllPortsSameDT=off  OutDataTypeStr=boolean
  AND2 : Logic  IconShape=distinctive  AllPortsSameDT=off  OutDataTypeStr=boolean
  Carrier1 : simulink/Sources/Repeating Sequence  rep_seq_t=[0 Ts/2 Ts]  rep_seq_y=[0 Ts-(1e-16) 0]
  Carrier2 : simulink/Sources/Repeating Sequence  rep_seq_t=[0 Ts/2 Ts]  rep_seq_y=[Ts-(1e-16) 0 Ts-(1e-16)]
  Constant : Constant
  Constant1 : Constant  Value=2
  Constant2 : Constant  Value=3
  Demux : Demux  Outputs=3
  GreaterThan{,1..3} (4 alike) : RelationalOperator  OutDataTypeStr=boolean  RndMeth=Simplest
  GreaterThan4 : RelationalOperator  Operator===  OutDataTypeStr=boolean  RndMeth=Simplest
  GreaterThan5 : RelationalOperator  Operator===  OutDataTypeStr=boolean  RndMeth=Simplest
  GreaterThan6 : RelationalOperator  Operator===  OutDataTypeStr=boolean  RndMeth=Simplest
  MATLAB Function : MATLAB Function  TreatAsAtomicUnit=on
  XOR : Logic  Operator=XOR  IconShape=distinctive  AllPortsSameDT=off  OutDataTypeStr=boolean
  XOR1 : Logic  Operator=XOR  IconShape=distinctive  AllPortsSameDT=off  OutDataTypeStr=boolean
  XOR2 : Logic  Operator=XOR  IconShape=distinctive  AllPortsSameDT=off  OutDataTypeStr=boolean
  Gate 1 Pulse : Outport
  Gate 3 Pulse : Outport  Port=2
  Gate 5 Pulse : Outport  Port=3
  wires:
  Carrier1/1 -> GreaterThan/2, GreaterThan1/2, GreaterThan2/2
  MATLAB Function/2(S3) -> GreaterThan1/1
  XOR/1 -> Gate 1 Pulse/1
  MATLAB Function/3(S5) -> GreaterThan2/1
  Constant/1 -> GreaterThan4/1
  MATLAB Function/4(addtime) -> GreaterThan3/1
  GreaterThan/1 -> XOR/1
  AND1/1 -> XOR1/2
  GreaterThan3/1 -> AND/1, AND1/1, AND2/1
  GreaterThan1/1 -> XOR1/1
  XOR2/1 -> Gate 5 Pulse/1
  GreaterThan4/1 -> AND/2
  MATLAB Function/1(S1) -> GreaterThan/1
  Carrier2/1 -> GreaterThan3/2
  GreaterThan2/1 -> XOR2/1
  GreaterThan5/1 -> AND1/2
  Constant2/1 -> GreaterThan6/1
  "S1, S3, S5"/1 -> Demux/1
  AND/1 -> XOR/2
  AND2/1 -> XOR2/2
  Constant1/1 -> GreaterThan5/1
  XOR1/1 -> Gate 3 Pulse/1
  MATLAB Function/5(addidx) -> GreaterThan6/2, GreaterThan5/2, GreaterThan4/2
  Demux/3 -> MATLAB Function/3("S5 ")
  Demux/1 -> MATLAB Function/1("S1 ")
  Demux/2 -> MATLAB Function/2("S3 ")
  GreaterThan6/1 -> AND2/2

== matlab function NN Controlled IM Drive/Space Vector PWM based VSI /Gating Pulse Generator/Gate Pulse Generator for 7212 Sequence/For Even Sector/MATLAB Function1 ==
  data: S1 input; S1 output; S3 input; S5 input; S3 output; S5 output; subtime output; subidx output
function [S1, S3, S5, subtime,subidx] = fcn(S1, S3, S5)
    S = [S1 S3 S5];
    [~, idx] = mink([S1 S3 S5], 3);
    
    S(idx(2)) = (S(idx(2)) + S(idx(3)))/2;
    
    subidx = idx(2);
    subtime = S(idx(3)) - S(idx(2));
    
    S1 = S(1);
    S3 = S(2);
    S5 = S(3);
end

== matlab function NN Controlled IM Drive/Space Vector PWM based VSI /Gating Pulse Generator/Gate Pulse Generator for 0121 Sequence/For Even Sector/MATLAB Function ==
  data: S1 input; S1 output; S3 input; S5 input; S3 output; S5 output; addtime output; addidx output
function [S1, S3, S5, addtime,addidx] = fcn(S1, S3, S5)
    S = [S1 S3 S5];
    [~, idx] = mink([S1 S3 S5], 3);
    
    addtime = (S(idx(2)) - S(idx(1)))/2;
    addidx = idx(2);
    S(idx(2)) = S(idx(2)) - addtime;
    
    S1 = S(1);
    S3 = S(2);
    S5 = S(3);
end

== matlab function NN Controlled IM Drive/Space Vector PWM based VSI /Switching Times and Sector/Switch Times and Sequence Calculation ==
  data: Vref input; angle input; Ts input; Vbus input; sector output
function sector  = fcn(Vref, angle, Ts, Vbus)
    
    numzones = 3;
    %     Using ML Models 
    m = (2/sqrt(3))*(Vref/Vbus);
    theta = rem(angle, (pi/3));
    flag = 0;
    if numzones == 1
        flag = 1;
    end
    
    %Switching times calculation of different vectors
    if m <= 1                % Linear modulation (Overmodulation mode 0)
        n2 = Vref*cos( theta );
        n1 = Vref*cos( (pi/3) - theta );

        T1 = (2*Ts/(3*Vbus)) * ((-n1) + (2*n2));
        T2 = (2*Ts/(3*Vbus)) * ((2*n1) - n2);
        T0 = Ts-(T1+T2);
        flag = 1;
        
    elseif m<=1.05      % Overmodulation mode I
        alpha_t = (pi/6) - acos(1/m);
        alpha_t = alpha_t/2;
        if theta > alpha_t && theta < (pi/3) - alpha_t
            T1 = (sin( (pi/3) - theta ) / ( sin( (pi/3) - theta ) + sin( theta ) ) ) * Ts;
            T2 = Ts-T1;
            T0=0;
        else
            n2 = Vref*cos( theta );
            n1 = Vref*cos( (pi/3) - theta );
            T1 = (2*Ts/(3*Vbus)) * ((-n1) + (2*n2));
            T2 = (2*Ts/(3*Vbus)) * ((2*n1) - n2);
            T0 = Ts-(T1+T2);
            flag = 1;
        end
        
    elseif m <= 1.10    % Overmodulation mode II
        alpha_h = (pi/6) - acos(1/m);
        if theta <= alpha_h
            T1 = Ts;
            T2=0;
            T0=0;
            
        elseif theta > alpha_h && theta < (pi/3) - alpha_h
            T1 = (sin( (pi/3) - theta ) / ( sin( (pi/3) - theta ) + sin( theta ) ) ) * Ts;
            T2 = Ts-T1;
            T0=0;
            
        else
            T1 = 0;
            T2 = Ts;
            T0 = 0;
        end
        
    else        % Six Step Mode
        if theta <= (pi/6)
            T1 = Ts;
            T2 = 0;
            T0 = 0;
        else
            T1 = 0;
            T2 = Ts;
            T0 = 0;
        end
        
    end
    
    if flag == 1
        % Switching Sequence Determination
        Q1 = (cos(theta) - (Vref/Vbus)) * T1;
        Q2 = (cos( (pi/3) - theta) - (Vref/Vbus)) * T2;
        Q0 = - (Vref/Vbus)*T0;
        D = sin(theta) * T1;

        %Error Functions (Squared) for Different Switching Sequences
        F_0127 = ( (1/3) * ( (0.5*Q0).^2 ) * T0 / (2*Ts) ) + ( (1/3) * ( ( (0.5*Q0).^2 ) + ( 0.5*Q0* ( (0.5*Q0) + Q1 ) ) + ( ( 1* ( (0.5*Q0) + Q1 ) ).^2) ) * (T1/Ts) ) + ( (1/3) * ( ( ( (0.5*Q0) + Q1).^2) - ( ( (0.5*Q0) + Q1) * (0.5*Q0) ) + ( (0.5*Q0).^2 ) ) * (T2/Ts) ) + ( (1/3) * ( (0.5*Q0).^2 ) * ( T0 / (2*Ts) ) ) + ( (1/3) * (D.^2) * ( (T1+T2) / Ts ) );

        F_012 = ( (4/27) * (Q0.^2) * (T0/Ts) ) + ( (4/27) * ( (Q0.^2) + ( Q0*(Q0+Q1) ) + ( (Q0+Q1).^2 ) ) * (T1/Ts) ) + ( (4/27) * ( (Q0+Q1).^2 ) * (T2/Ts) ) + ( (4/27) * (D.^2) * ( (T1+T2) / Ts) );

        F_721 = ( (4/27) * (Q0.^2) * (T0/Ts) ) + ( (4/27) * ( (Q0.^2) + ( Q0*(Q0+Q2) ) + ( (Q0+Q2).^2 ) ) * (T2/Ts) ) + ( (4/27) * ( (Q0+Q2).^2 ) * (T1/Ts) ) + ( (4/27) * (D.^2) * ( (T1+T2) / Ts) );

        F_0121 = ( (1/3) * (Q0.^2) * (T0/Ts) ) + ( (1/3) * ( (Q0.^2) + ( Q0*( Q0 + (0.5*Q1) ) ) + ( ( Q0 + (0.5*Q1) ).^2 ) ) * ( T1 / (2*Ts) ) ) + ( (1/3) * ( ( ( Q0 + (0.5*Q1) ).^2 ) - ( ( Q0 + (0.5*Q1) ) * (0.5*Q1) ) + ( (0.5*Q1).^2 ) ) * (T2/Ts) ) + ( (1/3) * ( (0.5*Q1).^2 ) * (T1 / (2*Ts) ) ) + ( (1/3) * ( (0.5*D).^2 ) * ( (T1+T2) / Ts ) );

        F_7212 = ( (1/3) * (Q0.^2) * (T0/Ts) ) + ( (1/3) * ( (Q0.^2) + ( Q0*( Q0 + (0.5*Q2) ) ) + ( ( Q0 + (0.5*Q2) ).^2 ) ) * ( T2 / (2*Ts) ) ) + ( (1/3) * ( ( ( Q0 + (0.5*Q2) ).^2 ) - ( ( Q0 + (0.5*Q2) ) * (0.5*Q2) ) + ( (0.5*Q2).^2 ) ) * (T1/Ts) ) + ( (1/3) * ( (0.5*Q2).^2 ) * (T2 / (2*Ts) ) ) + ( (1/3) * ( (0.5*D).^2 ) * ( (T1+T2) / Ts ) );

        F_1012 = ( (1/3) * ( ( 0.5*Q1).^2 ) * (T1 / (2*Ts) ) ) + ( (1/3) * ( ( (0.5*Q1).^2 ) + ( 0.5*Q1*( (0.5*Q1) + Q0 ) ) + ( ( (0.5*Q1) + Q0 ).^2 ) ) * (T0/Ts) ) + ( (1/3) * ( ( ( (0.5*Q1) + Q0 ).^2 ) - ( ( (0.5*Q1) + Q0 )*Q2 ) + (Q2.^2) ) * ( T1 / (2*Ts) ) ) + ( (1/3) * (Q2.^2) * (T2/Ts) ) + ( (1/3) * ( (0.5*D).^2 ) * ( T1 / (2*Ts) ) ) + ( ( (0.5*D).^2 ) * (T0/Ts) ) + ( (1/3) * ( ( (0.5*D).^2 ) + ( (0.5*D) * D ) + (D.^2) ) * ( T1 / (2*Ts) ) ) + ( (1/3) * (D.^2) * (T2/Ts) );

        F_2721 = ( (1/3) * ( ( 0.5*Q2).^2 ) * (T2 / (2*Ts) ) ) + ( (1/3) * ( ( (0.5*Q2).^2 ) + ( 0.5*Q2*( (0.5*Q2) + Q0 ) ) + ( ( (0.5*Q2) + Q0 ).^2 ) ) * (T0/Ts) ) + ( (1/3) * ( ( ( (0.5*Q2) + Q0 ).^2 ) - ( ( (0.5*Q2) + Q0 )*Q1 ) + (Q1.^2) ) * ( T2 / (2*Ts) ) ) + ( (1/3) * (Q1.^2) * (T1/Ts) ) + ( (1/3) * ( (0.5*D).^2 ) * ( T2 / (2*Ts) ) ) + ( ( (0.5*D).^2 ) * (T0/Ts) ) + ( (1/3) * ( ( (0.5*D).^2 ) + ( (0.5*D) * D ) + (D.^2) ) * ( T2 / (2*Ts) ) ) + ( (1/3) * (D.^2) * (T1/Ts) );
        
        if numzones == 1
            F = [F_0127];
            
        elseif numzones == 3
            %For Three Zone Hybrid PWM
            F = [F_0127, F_0121, F_7212];
            
        elseif numzones == 5
            %For Five Zone Hybrid PWM
            F = [F_0127, F_0121, F_7212, F_1012, F_2721];
        
        elseif numzones == 7
            %For Seven Zone Hybrid PWM
            F = [F_0127, F_0121, F_7212, F_1012, F_2721, F_012, F_721];
            
        else
            F = F_0127;
        end
        
        [~, idx] = min(F);

        if idx == 1
            switchseq = "0127";
        elseif idx == 2
            switchseq = "0121";
        elseif idx == 3
            switchseq = "7212";
        elseif idx == 4
            switchseq = "1012";
        elseif idx == 5
            switchseq = "2721";
        elseif idx == 6
            switchseq = "012";
        elseif idx == 7
            switchseq = "721";
        else
            switchseq = "0127";
        end
        
    else
        if theta < (pi/6)
            switchseq = "0121";
        else
            switchseq = "7212";
        end
    end
    
    % Switching Times calculation of switches
    Vsamp = Vref*exp(1i*angle);
    
    V1 = Vbus*exp(1i*0);
    V2 = Vbus*exp(1i*(pi/3));
    V3 = Vbus*exp(1i*(2*pi/3));
    V4 = Vbus*exp(1i*(3*pi/3));
    V5 = Vbus*exp(1i*(4*pi/3));
    V6 = Vbus*exp(1i*(5*pi/3));

    V = [V1; V2; V3; V4; V5; V6];
    V = V - Vsamp;
    [~, minVidx] = mink(V, 2);

%         minVidx = minVidx(:, 1);

    if max(minVidx) == 6 && min(minVidx) == 1
        minVidx = 6;
    else
        minVidx = min(minVidx);
    end
    
    sector = minVidx;
    
    if switchseq == "0127"
        swseq = 1;
    elseif switchseq == "0121"
        swseq = 2;
    elseif switchseq == "7212"
        swseq = 3;
    elseif switchseq == "1012"
        swseq = 4;
    elseif switchseq == "2721"
        swseq = 5;
    elseif switchseq == "012"
        swseq = 6;
    elseif switchseq == "721"
        swseq = 7;
    else
        swseq = 1;
    end
%     
%     %Using NN to predict switch times
%     
%     %Loading Necessary weight matrices
%     W1 = evalin('base', 'W1R');
%     b1 = evalin('base', 'b1R');
%     W2 = evalin('base', 'W2R');
%     b2 = evalin('base', 'W2R');
%     
%     %Predicting Switch Times
%     X = [m angle];
% %     y1 = zeros(1, size(b1, 1));
% %     y2 = zeros(1, size(b2, 2));
%     
%     y = X*(W1');
%     y = y + b1';      %Passing through 1st Layer (Hidden)
%     y = tanh(y);                  %Applying Activation Function (tanh)
%     
%     y = y*W2';
%     y = y+b2';        %Passing through 2nd Layer (Output)
%     y = 1./(1+exp(-y));      %Applying Activation Function (sigmoid)
%     
%     %Allocating Switch Times
%     S1 = y(1)*Ts;
%     S3 = y(2)*Ts;
%     S5 = y(3)*Ts;
    
end

== matlab function NN Controlled IM Drive/Space Vector PWM based VSI /Gating Pulse Generator/Gate Pulse Generator for 1012 Sequence/For Even Sector/MATLAB Function1 ==
  data: S1 input; S1 output; S3 input; S5 input; S3 output; S5 output; subtime output; subidx output
function [S1, S3, S5, subtime,subidx] = fcn(S1, S3, S5)
    S = [S1 S3 S5];
    [~, idx] = mink([S1 S3 S5], 3);
    
    subtime = ( ( S(idx(2)) - S(idx(1)) )/2);
    S(idx(1)) = S(idx(1)) + subtime;
    subidx = idx(1);
    
    S1 = S(1);
    S3 = S(2);
    S5 = S(3);
end

== matlab function NN Controlled IM Drive/Space Vector PWM based VSI /Gating Pulse Generator/Gate Pulse Generator for 0127 Sequence 1/For Even Sector/MATLAB Function ==
  data: S1 input; S1 output; S3 input; S5 input; S3 output; S5 output; addtime output; addidx output
function [S1, S3, S5, addtime,addidx] = fcn(S1, S3, S5)
    S = [S1 S3 S5];
    [~, idx] = mink([S1 S3 S5], 3);
    
    addtime = (S(idx(3)) - S(idx(2)))/2;
    addidx = idx(3);
    S(idx(3)) = S(idx(3)) - addtime;
    
    S1 = S(1);
    S3 = S(2);
    S5 = S(3);
end

== matlab function NN Controlled IM Drive/Space Vector PWM based VSI /Gating Pulse Generator/Gate Pulse Generator for 0121 Sequence/For Odd Sector/MATLAB Function ==
  data: S1 input; S1 output; S3 input; S5 input; S3 output; S5 output; subtime output; subidx output
function [S1, S3, S5, subtime,subidx] = fcn(S1, S3, S5)
    S = [S1 S3 S5];
    [~, idx] = mink([S1 S3 S5], 3);
    
    S(idx(2)) = (S(idx(2)) + S(idx(3)))/2;
    
    subidx = idx(2);
    subtime = S(idx(3)) - S(idx(2));
    
    S1 = S(1);
    S3 = S(2);
    S5 = S(3);
end

== matlab function NN Controlled IM Drive/Space Vector PWM based VSI /MATLAB Function ==
  data: angle input; angle_conv output
function angle_conv = fcn(angle)
    if angle<0
        angle_conv=(2*pi)+angle;
    else
        angle_conv=angle;
    end
%     angle_conv = rem(angle_conv + (time*ws), 2*pi);
end

== matlab function NN Controlled IM Drive/Space Vector PWM based VSI /Gating Pulse Generator/Gate Pulse Generator for 1012 Sequence/For Odd Sector/MATLAB Function ==
  data: S1 input; S1 output; S3 input; S5 input; S3 output; S5 output; addtime output; addidx output
function [S1, S3, S5, addtime,addidx] = fcn(S1, S3, S5)
    S = [S1 S3 S5];
    [~, idx] = mink([S1 S3 S5], 3);
    
    addtime = (S(idx(3)) - S(idx(2)))/2;
    addidx = idx(3);
    S(idx(3)) = S(idx(3)) - addtime;
    
    S1 = S(1);
    S3 = S(2);
    S5 = S(3);
end

== matlab function NN Controlled IM Drive/Space Vector PWM based VSI /Gating Pulse Generator/Gate Pulse Generator for 2721 Sequence/For Even Sector/MATLAB Function ==
  data: S1 input; S1 output; S3 input; S5 input; S3 output; S5 output; addtime output; addidx output
function [S1, S3, S5, addtime,addidx] = fcn(S1, S3, S5)
    S = [S1 S3 S5];
    [~, idx] = mink([S1 S3 S5], 3);
    
    addtime = (S(idx(3)) - S(idx(2)))/2;
    addidx = idx(3);
    S(idx(3)) = S(idx(3)) - addtime;
    
    S1 = S(1);
    S3 = S(2);
    S5 = S(3);
end

== matlab function NN Controlled IM Drive/Space Vector PWM based VSI /Switching Times and Sector/MATLAB Function1 ==
  data: u input; S1 output; S3 output; S5 output
function [S1, S3, S5] = fcn(u)
    S1 = u(1);
    S3 = u(2);
    S5 = u(3);
end

== matlab function NN Controlled IM Drive/Space Vector PWM based VSI /Gating Pulse Generator/Gate Pulse Generator for 7212 Sequence/For Odd Sector/MATLAB Function ==
  data: S1 input; S1 output; S3 input; S5 input; S3 output; S5 output; addtime output; addidx output
function [S1, S3, S5, addtime,addidx] = fcn(S1, S3, S5)
    S = [S1 S3 S5];
    [~, idx] = mink([S1 S3 S5], 3);
    
    addtime = (S(idx(2)) - S(idx(1)))/2;
    addidx = idx(2);
    S(idx(2)) = S(idx(2)) - addtime;
    
    S1 = S(1);
    S3 = S(2);
    S5 = S(3);
end

== matlab function NN Controlled IM Drive/Space Vector PWM based VSI /Gating Pulse Generator/Gate Pulse Generator for 2721 Sequence/For Odd Sector/MATLAB Function1 ==
  data: S1 input; S1 output; S3 input; S5 input; S3 output; S5 output; subtime output; subidx output
function [S1, S3, S5, subtime,subidx] = fcn(S1, S3, S5)
    S = [S1 S3 S5];
    [~, idx] = mink([S1 S3 S5], 3);
    
    subtime = ( ( S(idx(2)) - S(idx(1)) )/2);
    S(idx(1)) = S(idx(1)) + subtime;
    subidx = idx(1);
    
    S1 = S(1);
    S3 = S(2);
    S5 = S(3);
end

== matlab function NN Controlled IM Drive/Space Vector PWM based VSI /Switching Times and Sector/Feature Expand ==
  data: X input; new_X output size=[1 18]
function new_X = fcn(X)
    X = X';
    new_X = zeros(1,18);
    new_X(1, 1) = X(1, 1);
    new_X(1, 2) = X(1, 2);
    
    %Include sinusoidal terms (1st order)
    new_X(1, 3) = sin(X(1, 1));
    new_X(1, 4) = sin(X(1, 2));
    new_X(1, 5) = cos(X(1, 1));
    new_X(1, 6) = cos(X(1, 2));
%     new_X(1, 7) = sin(X(1, 1).*X(1, 2));
%     new_X(1, 8) = cos(X(1, 1).*X(1, 2));
    
%Include 2nd harmonic sinusoidal terms
    new_X(1, 7) = sin(2*X(1, 1));
    new_X(1, 8) = sin(2*X(1, 2));
    new_X(1, 9) = cos(2*X(1, 1));
    new_X(1, 10) = cos(2*X(1, 2));
    
        %Include 3rd harmonic sinusoidal terms
    new_X(1, 11) = sin(3*X(1, 1));
    new_X(1, 12) = sin(3*X(1, 2));
    new_X(1, 13) = cos(3*X(1, 1));
    new_X(1, 14) = cos(3*X(1, 2));
    
    %Include 4th harmonic sinusoidal terms
    new_X(1, 15) = sin(4*X(1, 1));
    new_X(1, 16) = sin(4*X(1, 2));
    new_X(1, 17) = cos(4*X(1, 1));
    new_X(1, 18) = cos(4*X(1, 2));

%     %Include 2nd order terms
%     new_X(:, 3) = X(:, 1).*X(:, 1);
%     new_X(:, 4) = X(:, 1).*X(:, 2);
%     new_X(:, 5) = X(:, 2).*X(:, 2);
    
%     %Include 3rd order terms
%     new_X(:, 6) = X(:, 1).*X(:, 1).*X(:, 1);
%     new_X(:, 7) = X(:, 1).*X(:, 1).*X(:, 2);
%     new_X(:, 8) = X(:, 1).*X(:, 2).*X(:, 2);
%     new_X(:, 9) = X(:, 2).*X(:, 2).*X(:, 2);
%     
%     %Incluce 4th order terms
%     new_X(:, 10) = X(:, 1).*X(:, 1).*X(:, 1).*X(:, 1);
%     new_X(:, 11) = X(:, 1).*X(:, 1).*X(:, 1).*X(:, 2);
%     new_X(:, 12) = X(:, 1).*X(:, 1).*X(:, 2).*X(:, 2);
%     new_X(:, 13) = X(:, 1).*X(:, 2).*X(:, 2).*X(:, 2);
%     new_X(:, 14) = X(:, 2).*X(:, 2).*X(:, 2).*X(:, 2);
%     
%     %Incluce 5th order terms
%     new_X(:, 15) = X(:, 1).*X(:, 1).*X(:, 1).*X(:, 1).*X(:, 1);
%     new_X(:, 16) = X(:, 1).*X(:, 1).*X(:, 1).*X(:, 1).*X(:, 2);
%     new_X(:, 17) = X(:, 1).*X(:, 1).*X(:, 1).*X(:, 2).*X(:, 2);
%     new_X(:, 18) = X(:, 1).*X(:, 1).*X(:, 2).*X(:, 2).*X(:, 2);
%     new_X(:, 19) = X(:, 1).*X(:, 2).*X(:, 2).*X(:, 2).*X(:, 2);
%     new_X(:, 20) = X(:, 2).*X(:, 2).*X(:, 2).*X(:, 2).*X(:, 2);
%     
%     %Incluce 6th order terms
%     new_X(:, 21) = X(:, 1).*X(:, 1).*X(:, 1).*X(:, 1).*X(:, 1).*X(:, 1);
%     new_X(:, 22) = X(:, 1).*X(:, 1).*X(:, 1).*X(:, 1).*X(:, 1).*X(:, 2);
%     new_X(:, 23) = X(:, 1).*X(:, 1).*X(:, 1).*X(:, 1).*X(:, 2).*X(:, 2);
%     new_X(:, 24) = X(:, 1).*X(:, 1).*X(:, 1).*X(:, 2).*X(:, 2).*X(:, 2);
%     new_X(:, 25) = X(:, 1).*X(:, 1).*X(:, 2).*X(:, 2).*X(:, 2).*X(:, 2);
%     new_X(:, 26) = X(:, 1).*X(:, 2).*X(:, 2).*X(:, 2).*X(:, 2).*X(:, 2);
%     new_X(:, 27) = X(:, 2).*X(:, 2).*X(:, 2).*X(:, 2).*X(:, 2).*X(:, 2);
end

== matlab function NN Controlled IM Drive/Space Vector PWM based VSI /Switching Times and Sector/m ==
  data: Vref input; m output; Vbus input
function m = fcn(Vref, Vbus)
    m = (2/sqrt(3)) * Vref/Vbus;
end

== matlab function NN Controlled IM Drive/Space Vector PWM based VSI /Switching Times and Sector/Angle Calculation1/MATLAB Function ==
  data: wold input; wnew output; wTs input
function wnew = fcn(wold, wTs)
    wnew = rem(wold + wTs, 2*pi);
end
